simulink model "Fbridge_sim"  (R2023a)
settings: Solver=VariableStepAuto  StartTime=0.0  StopTime=20  MaxStep=1e-4  RelTol=1e-4  EnableMultiTasking=on
undefined symbols (not defined in the file or in its folder): D
libraries: spsMosfetLib x12, simulink x5, spsDCVoltageSourceLib x3, spsDCMachineLib x2, spsSeriesRLCBranchLib x2, spspowerguiLib x2, spsControlledVoltageSourceLib x1
settings Model: Creator=The MathWorks, Inc.  LastModifiedBy=Admin
settings SolverCC: AlgebraicLoopSolver=TrustRegion
settings DataIOCC: LimitDataPoints=on  SaveFormat=Array  ReturnWorkspaceOutputs=off
settings OptimizationCC: ExpressionDepthLimit=2147483647  InitFltsAndDblsToZero=on  LifeSpan=inf
settings DebuggingCC: SaveWithParameterizedLinksMsg=none  UnderspecifiedInitializationDetection=Classic  MergeDetectMultiDrivingBlocksExec=none  SignalResolutionControl=TryResolveAllWithWarning  SolverPrmCheckMsg=warning  MultiTaskDSMMsg=warning  MultiTaskCondExecSysMsg=none  FcnCallInpInsideContextMsg=warning  UnconnectedInputMsg=warning  UnconnectedOutputMsg=warning  UnconnectedLineMsg=warning  StateNameClashWarn=warning  SFUnexpectedBacktrackingDiag=warning  SFNoUnconditionalDefaultTransitionDiag=warning  SFExecutionAtInitializationDiag=none  ArithmeticOperatorsInVariantConditions=warning
settings HardwareCC: ProdBitPerPointer=32  ProdBitPerSizeT=32  ProdBitPerPtrDiffT=32  ProdLargestAtomicFloat=None  ProdIntDivRoundTo=Undefined  ProdEndianess=Unspecified  ProdWordSize=32  ProdHWDeviceType=32-bit Generic
settings ModelReferenceCC: EnableRefExpFcnMdlSchedulingChecks=on  PropagateSignalLabelsOutOfModel=off
settings SFSimCC: SimUseLocalCustomCode=off  CustomCodeUndefinedFunction=UseInterfaceOnly
settings RTWCC: RTWUseLocalCustomCode=off  DLArmComputeVersion=19.05
settings CodeAppCC: StateflowObjectComments=on
settings GRTTargetCC: TargetFcnLib=ansi_tfl_tmw.mat  TargetLangStandard=C89/C90 (ANSI)  CombineOutputUpdateFcns=off  GRTInterface=on
settings ConfigComp: CovMetricSettings=dw  CovSaveCumulativeToWorkspaceVar=on  CovSaveSingleToWorkspaceVar=on  CovExternalEMLEnable=off  CovSFcnEnable=off
settings SimscapeCC: SimscapeNormalizeSystem=off  SimscapeNominalValues={1, 'bar'; 1, 'cm^3/s'; 1, 'bar*kg/s'; 1, 'kJ/kg'; 1, 'kW'; }

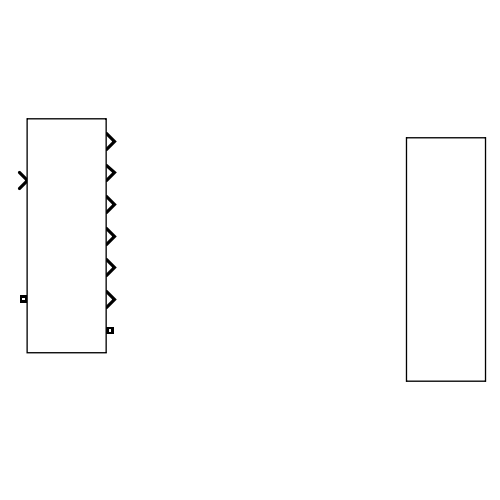
[thumbnail: Simulink's stored preview of the top-level diagram]
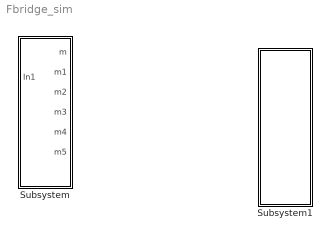
== system Fbridge_sim ==
  Subsystem : Subsystem
  Subsystem1 : Subsystem

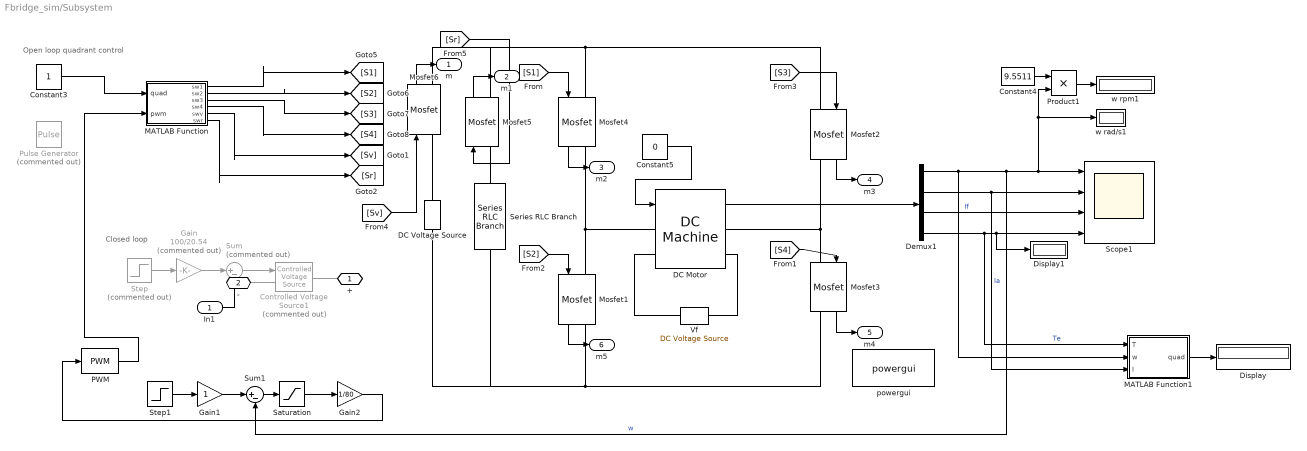
== system Fbridge_sim/Subsystem ==
  note: Open loop quadrant control
  note: Closed loop
  In1 : Inport
  Constant3 : Constant
  Constant4 : Constant  Value=9.5511
  Constant5 : Constant  Value=0
  Controlled Voltage Source1 : spsControlledVoltageSourceLib/Controlled Voltage Source  Commented=on  Initialize=on  Source_Type=DC  Amplitude=0  Phase=0  Frequency=0  Measurements=None
  DC Motor : spsDCMachineLib/DC Machine  PresetModel=No  MechanicalLoad=Torque TL  FieldType=Wound  ShowDetailedParameters=on  MeasurementBus=off  RLa=[2.581 0.028]  RLf=[2.02 0.128]  Laf=0.1  MachineConstant=Torque constant (N.m/A)  Ke=1.8  Kt=1.8  J=0.01  Bm=0.0006  Tf=0  w0=0  Ifinit=2.47524752475248  TsPowergui=0  TsBlock=-1
  DC Voltage Source : spsDCVoltageSourceLib/DC Voltage Source  Amplitude=80  Measurements=None
  Demux1 : Demux
  Display : Display
  Display1 : Display
  Gain : Gain  Commented=on  Gain=100/20.54
  Gain1 : Gain
  Gain2 : Gain  Gain=1/80
  MATLAB Function : MATLAB Function  TreatAsAtomicUnit=on
  MATLAB Function1 : MATLAB Function  TreatAsAtomicUnit=on
  Mosfet{1..6} (6 alike) : spsMosfetLib/Mosfet  Ron=0.1  Lon=0  Rd=0.01  Vfd=0  IC=0  Rs=1e5  Cs=inf  Measurements=on
  PWM : simulink/Discontinuities/PWM  DisableCoverage=on  Period=0.0001  InitialDelay=0  DisallowZeroDutyCycle=off  RunAtFixedTimeIntervals=off  SampleTime=0.1
  Product1 : Product
  Pulse Generator : DiscretePulseGenerator  Commented=on  PulseType=Time based  Period=0.0001  PulseWidth=D
  Saturation : Saturate  UpperLimit=80  LowerLimit=0
  Scope1 : Scope  NumInputPorts=4
  Series RLC Branch : spsSeriesRLCBranchLib/Series RLC Branch  LConnTagsString=__new0  RConnTagsString=__new0  BranchType=R  Resistance=10  Inductance=1e-3  SetiL0=off  InitialCurrent=0  Capacitance=1e-6  Setx0=off  InitialVoltage=0  Measurements=None
  Step : Step  Commented=on  After=100  SampleTime=0
  Step1 : Step  After=200  SampleTime=0
  Sum : Sum  Commented=on  Inputs=|+-
  Sum1 : Sum  Inputs=|+-
  Vf : spsDCVoltageSourceLib/DC Voltage Source  Amplitude=5  Measurements=None
  powergui : spspowerguiLib/powergui  SimulationMode=Discrete  SampleTime=20e-6  frequency=60  Iterations=50  frequencyindice=0  Pbase=100e6  ErrMax=1e-4  UnitsV=kV  UnitsW=MW  buscounter=0  FunctionMessages=off  echomessages=off  EnableUseOfTLC=off  CurrentSourceSwitches=off  DisableSnubberDevices=off  DisableRonSwitches=off  DisableVfSwitches=off  DisplayEquations=off  AutomaticDiscreteSolvers=off  SolverType=Tustin/Backward Euler (TBE)  Interpol=off  ExternalGateDelay=off  methode=off  Ts=100  x0status=blocks  SPID=on  SwTol=0  HookPort=off  NonlinearTolerance=1e-4  nMaxIteration=100  ContinueOnMaxIteration=off  RestoreLinks=warning  ResistiveCurrentMeasurement=off  Frange=[0:2:500]  Ylog=off  Xlog=on  ShowGrid=off  save=off  variable=ZData  structure=0  ZoomFFT=on  StartTime=0.0  cycles=1  DisplayStyle=1  fundamental=60  FreqAxis=off  MaxFrequency=1000  frequencyindicesteady=1  RmsSteady=1  display=off
  w rad/s1 : Display
  w rpm1 : Display
  + : PMIOPort  Side=Right
  - : PMIOPort  Port=2  Side=Left
  m : Outport
  m1 : Outport  Port=2
  m2 : Outport  Port=3
  m3 : Outport  Port=4
  m4 : Outport  Port=5
  m5 : Outport  Port=6
  wires:
  PWM/1 -> MATLAB Function/2(pwm)
  [S4] -> Mosfet3/1
  Mosfet4/1 -> m2/1
  MATLAB Function/1(sw1) -> [S1]
  Gain/1 -> Sum/1
  Demux1/3 -> Scope1/3  "If"
  Demux1/2 -> MATLAB Function1/3(I), Scope1/2  "Ia"
  Demux1/1 -> MATLAB Function1/2(w), Sum1/2, Scope1/1, Product1/2, w rad/s1/1  "w"
  DC Motor/1 -> Demux1/1
  Saturation/1 -> Gain2/1
  [Sr] -> Mosfet5/1
  [S1] -> Mosfet4/1
  In1/1 -> Sum/2
  Demux1/4 -> MATLAB Function1/1(T), Display1/1, Scope1/4  "Te"
  Mosfet3/1 -> m4/1
  Mosfet6/1 -> m/1
  [Sv] -> Mosfet6/1
  [S3] -> Mosfet2/1
  Sum/1 -> Controlled Voltage Source1/1
  [S2] -> Mosfet1/1
  Constant4/1 -> Product1/1
  Constant5/1 -> DC Motor/1
  MATLAB Function/3(sw3) -> [S3]
  Constant3/1 -> MATLAB Function/1(quad)
  Step1/1 -> Gain1/1
  MATLAB Function1/1(quad) -> Display/1
  MATLAB Function/5(swv) -> [Sv]
  MATLAB Function/6(swr) -> [Sr]
  MATLAB Function/2(sw2) -> [S2]
  MATLAB Function/4(sw4) -> [S4]
  Product1/1 -> w rpm1/1
  Sum1/1 -> Saturation/1
  Gain2/1 -> PWM/1
  Step/1 -> Gain/1
  Gain1/1 -> Sum1/1
  Mosfet1/1 -> m5/1
  Mosfet5/1 -> m1/1
  Mosfet2/1 -> m3/1
  connections:
  Mosfet4/LConn1 -- Mosfet5/RConn1 -- Mosfet6/RConn1 -- Mosfet2/LConn1
  Series RLC Branch/LConn1 -- Mosfet5/LConn1
  Mosfet4/RConn1 -- DC Motor/LConn1 -- Mosfet1/LConn1
  Controlled Voltage Source1/LConn1 -- -/RConn1
  DC Motor/RConn2 -- Vf/LConn1
  Mosfet6/LConn1 -- DC Voltage Source/RConn1
  Mosfet1/RConn1 -- Series RLC Branch/RConn1 -- DC Voltage Source/LConn1 -- Mosfet3/RConn1
  DC Motor/LConn2 -- Vf/RConn1
  DC Motor/RConn1 -- Mosfet3/LConn1 -- Mosfet2/RConn1
  Controlled Voltage Source1/RConn1 -- +/RConn1

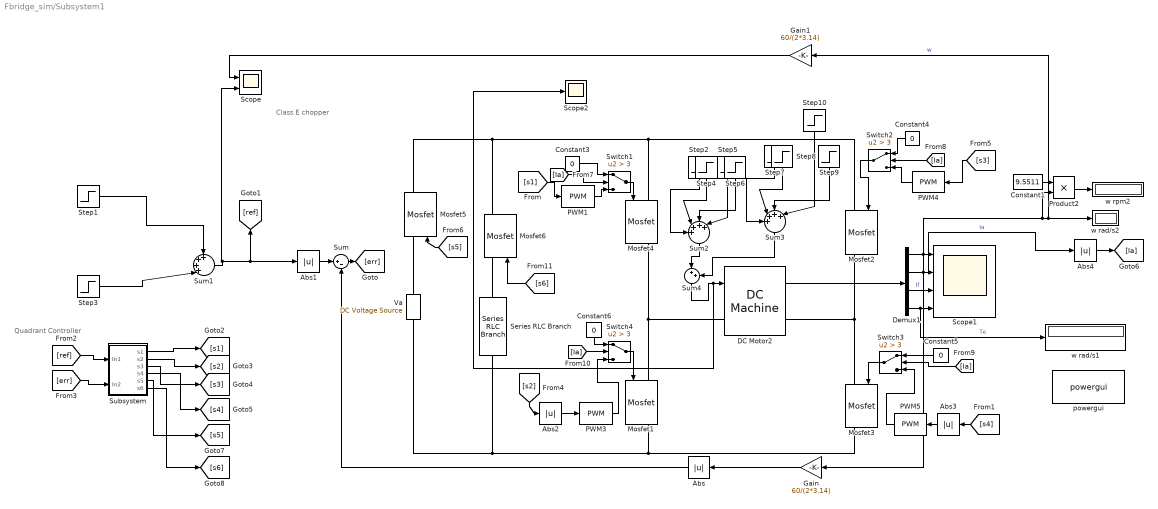
== system Fbridge_sim/Subsystem1 ==
  note: Quadrant Controller
  note: Class E chopper
  Abs{,1..4} (5 alike) : Abs  SaturateOnIntegerOverflow=off
  Constant1 : Constant  Value=9.5511
  Constant{3..6} (4 alike) : Constant  Value=0
  DC Motor2 : spsDCMachineLib/DC Machine  PresetModel=No  MechanicalLoad=Torque TL  FieldType=Permanent magnet  ShowDetailedParameters=on  MeasurementBus=off  RLa=[3 0.05]  RLf=[2.02 0.128]  Laf=0.1  MachineConstant=Back-emf constant (V/rpm)  Ke=0.029  Kt=0.27  J=0.012  Bm=0.0006  Tf=0.0958  w0=0  Ifinit=2.47524752475248  TsPowergui=0  TsBlock=-1
  Demux1 : Demux
  Gain : Gain  Gain=60/(2*3.14)
  Gain1 : Gain  Gain=60/(2*3.14)
  Mosfet{1..6} (6 alike) : spsMosfetLib/Mosfet  Ron=0.1  Lon=0  Rd=0.01  Vfd=0  IC=0  Rs=1e5  Cs=inf  Measurements=on
  PWM1 : simulink/Discontinuities/PWM  DisableCoverage=on  Period=1e-4  InitialDelay=0  DisallowZeroDutyCycle=off  RunAtFixedTimeIntervals=off  SampleTime=0.1
  PWM3 : simulink/Discontinuities/PWM  DisableCoverage=on  Period=5e-4  InitialDelay=0  DisallowZeroDutyCycle=off  RunAtFixedTimeIntervals=off  SampleTime=0.1
  PWM4 : simulink/Discontinuities/PWM  DisableCoverage=on  Period=1e-4  InitialDelay=0  DisallowZeroDutyCycle=off  RunAtFixedTimeIntervals=off  SampleTime=0.1
  PWM5 : simulink/Discontinuities/PWM  DisableCoverage=on  Period=5e-4  InitialDelay=0  DisallowZeroDutyCycle=off  RunAtFixedTimeIntervals=off  SampleTime=0.1
  Product2 : Product
  Scope : Scope  NumInputPorts=2
  Scope1 : Scope  NumInputPorts=4
  Scope2 : Scope
  Series RLC Branch : spsSeriesRLCBranchLib/Series RLC Branch  LConnTagsString=__new0  RConnTagsString=__new0  BranchType=R  Resistance=20  Inductance=1e-3  SetiL0=off  InitialCurrent=0  Capacitance=1e-6  Setx0=off  InitialVoltage=0  Measurements=None
  Step1 : Step  After=1000  SampleTime=0
  Step10 : Step  Time=17  After=-0.1  SampleTime=0
  Step2 : Step  Time=3  After=0.1  SampleTime=0
  Step3 : Step  Time=9  After=-2000  SampleTime=0
  Step4 : Step  Time=5  After=0.1  SampleTime=0
  Step5 : Step  Time=7  After=0.1  SampleTime=0
  Step6 : Step  Time=8  After=-0.3  SampleTime=0
  Step7 : Step  Time=12  After=-0.1  SampleTime=0
  Step8 : Step  Time=15  After=-0.1  SampleTime=0
  Step9 : Step  Time=18  After=+0.3  SampleTime=0
  Subsystem : Subsystem
  Sum : Sum  Inputs=|+-
  Sum1 : Sum  Inputs=++++|
  Sum2 : Sum  Inputs=++++|
  Sum3 : Sum  Inputs=++++|
  Sum4 : Sum  Inputs=|++
  Switch{1..4} (4 alike) : Switch  Criteria=u2 > Threshold  Threshold=3  SaturateOnIntegerOverflow=off  InputSameDT=off
  Va : spsDCVoltageSourceLib/DC Voltage Source  Amplitude=85  Measurements=None
  powergui : spspowerguiLib/powergui  SimulationMode=Discrete  SampleTime=20e-6  frequency=60  Iterations=50  frequencyindice=0  Pbase=100e6  ErrMax=1e-4  UnitsV=kV  UnitsW=MW  buscounter=0  FunctionMessages=off  echomessages=off  EnableUseOfTLC=off  CurrentSourceSwitches=off  DisableSnubberDevices=off  DisableRonSwitches=off  DisableVfSwitches=off  DisplayEquations=off  AutomaticDiscreteSolvers=off  SolverType=Tustin/Backward Euler (TBE)  Interpol=off  ExternalGateDelay=off  methode=off  Ts=100  x0status=blocks  SPID=on  SwTol=0  HookPort=off  NonlinearTolerance=1e-4  nMaxIteration=100  ContinueOnMaxIteration=off  RestoreLinks=warning  ResistiveCurrentMeasurement=off  Frange=[0:2:500]  Ylog=off  Xlog=on  ShowGrid=off  save=off  variable=ZData  structure=0  ZoomFFT=on  StartTime=0.0  cycles=1  DisplayStyle=1  fundamental=60  FreqAxis=off  MaxFrequency=1000  frequencyindicesteady=1  RmsSteady=1  display=off
  w rad/s1 : Display
  w rad/s2 : Display
  w rpm2 : Display
  wires:
  Demux1/4 -> w rad/s1/1, Scope1/4  "Te"
  DC Motor2/1 -> Demux1/1
  Demux1/2 -> Abs4/1, Scope1/2  "Ia"
  Demux1/3 -> Scope1/3  "If"
  Demux1/1 -> Gain1/1, w rad/s2/1, Product2/2, Gain/1, Scope1/1  "w"
  Constant1/1 -> Product2/1
  Product2/1 -> w rpm2/1
  [s2] -> Abs2/1
  [s3] -> PWM4/1
  Abs1/1 -> Sum/1
  [s1] -> PWM1/1
  Sum/1 -> [err]
  Subsystem/1(s1) -> [s1]
  Subsystem/2(s2) -> [s2]
  Subsystem/4(s4) -> [s4]
  Subsystem/3(s3) -> [s3]
  Step1/1 -> Sum1/1
  Sum1/1 -> Abs1/1, [ref], Scope/2
  [ref] -> Subsystem/1(In1)
  [err] -> Subsystem/2(In2)
  Abs2/1 -> PWM3/1
  Abs3/1 -> PWM5/1
  [s4] -> Abs3/1
  Step3/1 -> Sum1/4
  PWM1/1 -> Switch1/3
  Switch1/1 -> Mosfet4/1
  [Ia] -> Switch1/2
  Constant3/1 -> Switch1/1
  Gain/1 -> Abs/1
  Abs4/1 -> [Ia]
  PWM4/1 -> Switch2/3
  Constant4/1 -> Switch2/1
  [Ia] -> Switch2/2
  Switch2/1 -> Mosfet2/1
  Switch3/1 -> Mosfet3/1
  Constant5/1 -> Switch3/1
  [Ia] -> Switch3/2
  PWM5/1 -> Switch3/3
  PWM3/1 -> Switch4/3
  Constant6/1 -> Switch4/1
  [Ia] -> Switch4/2
  Switch4/1 -> Mosfet1/1
  [s5] -> Mosfet5/1
  Subsystem/5(s5) -> [s5]
  [s6] -> Mosfet6/1
  Gain1/1 -> Scope/1
  Abs/1 -> Sum/2
  Subsystem/6(s6) -> [s6]
  Step2/1 -> Sum2/1
  Step4/1 -> Sum2/2
  Step5/1 -> Sum2/4
  Step6/1 -> Sum2/3
  Sum2/1 -> Sum4/1
  Sum3/1 -> Sum4/2
  Sum4/1 -> Scope2/1, DC Motor2/1
  Step9/1 -> Sum3/3
  Step10/1 -> Sum3/4
  Step8/1 -> Sum3/2
  Step7/1 -> Sum3/1
  connections:
  Mosfet2/RConn1 -- Mosfet3/LConn1 -- DC Motor2/RConn1
  Mosfet4/RConn1 -- Mosfet1/LConn1 -- DC Motor2/LConn1
  Mosfet3/RConn1 -- Series RLC Branch/RConn1 -- Va/LConn1 -- Mosfet1/RConn1
  Mosfet4/LConn1 -- Mosfet5/RConn1 -- Mosfet6/RConn1 -- Mosfet2/LConn1
  Mosfet5/LConn1 -- Va/RConn1
  Mosfet6/LConn1 -- Series RLC Branch/LConn1

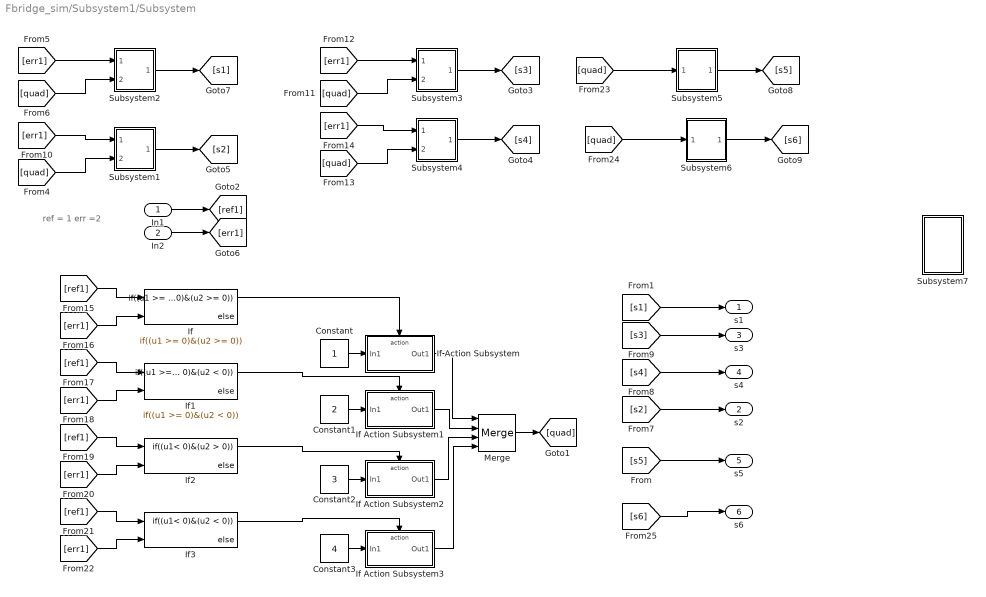
== system Fbridge_sim/Subsystem1/Subsystem ==
  note: ref = 1
      | err =2
  In1 : Inport
  In2 : Inport  Port=2
  Constant : Constant
  Constant1 : Constant  Value=2
  Constant2 : Constant  Value=3
  Constant3 : Constant  Value=4
  If : If  NumInputs=2  IfExpression=(u1 >= 0)&(u2 >= 0)
  If Action Subsystem : Subsystem  TreatAsAtomicUnit=on
  If Action Subsystem1 : Subsystem  TreatAsAtomicUnit=on
  If Action Subsystem2 : Subsystem  TreatAsAtomicUnit=on
  If Action Subsystem3 : Subsystem  TreatAsAtomicUnit=on
  If1 : If  NumInputs=2  IfExpression=(u1 >= 0)&(u2 < 0)
  If2 : If  NumInputs=2  IfExpression=(u1< 0)&(u2 > 0)
  If3 : If  NumInputs=2  IfExpression=(u1< 0)&(u2 < 0)
  Merge : Merge  Inputs=4
  Subsystem1 : Subsystem
  Subsystem2 : Subsystem
  Subsystem3 : Subsystem
  Subsystem4 : Subsystem
  Subsystem5 : Subsystem
  Subsystem6 : Subsystem
  Subsystem7 : Subsystem
  s1 : Outport
  s2 : Outport  Port=2
  s3 : Outport  Port=3
  s4 : Outport  Port=4
  s5 : Outport  Port=5
  s6 : Outport  Port=6
  wires:
  In1/1 -> [ref1]
  [s1] -> s1/1
  In2/1 -> [err1]
  [err1] -> Subsystem1/1(In1)
  [quad] -> Subsystem1/2(In2)
  Subsystem1/1(Out1) -> [s2]
  Subsystem2/1(Out1) -> [s1]
  [quad] -> Subsystem2/2(In2)
  [err1] -> Subsystem2/1(In1)
  [s3] -> s3/1
  [err1] -> Subsystem3/1(In1)
  [quad] -> Subsystem3/2(In2)
  Subsystem3/1(Out1) -> [s3]
  Subsystem4/1(Out1) -> [s4]
  [quad] -> Subsystem4/2(In2)
  [err1] -> Subsystem4/1(In1)
  [s2] -> s2/1
  [s4] -> s4/1
  [ref1] -> If/1
  [err1] -> If/2
  If/1 -> If Action Subsystem/Action
  If Action Subsystem/1(Out1) -> Merge/1
  Constant/1 -> If Action Subsystem/1(In1)
  Merge/1 -> [quad]
  [err1] -> If1/2
  [ref1] -> If1/1
  Constant1/1 -> If Action Subsystem1/1(In1)
  If Action Subsystem1/1(Out1) -> Merge/2
  If1/1 -> If Action Subsystem1/Action
  If2/1 -> If Action Subsystem2/Action
  [ref1] -> If2/1
  [err1] -> If2/2
  [err1] -> If3/2
  [ref1] -> If3/1
  If3/1 -> If Action Subsystem3/Action
  Constant2/1 -> If Action Subsystem2/1(In1)
  Constant3/1 -> If Action Subsystem3/1(In1)
  If Action Subsystem2/1(Out1) -> Merge/3
  If Action Subsystem3/1(Out1) -> Merge/4
  Subsystem5/1(Out1) -> [s5]
  [quad] -> Subsystem5/1(In2)
  [s5] -> s5/1
  [s6] -> s6/1
  [quad] -> Subsystem6/1(In2)
  Subsystem6/1(Out1) -> [s6]

== system Fbridge_sim/Subsystem1/Subsystem/If Action Subsystem ==
  In1 : Inport
  Action Port : ActionPort  ActionPortLabel=if((u1 >= 0)&(u2 >= 0))
  Out1 : Outport
  wires:
  In1/1 -> Out1/1

== system Fbridge_sim/Subsystem1/Subsystem/If Action Subsystem1 ==
  In1 : Inport
  Action Port : ActionPort  ActionPortLabel=if((u1 >= 0)&(u2 < 0))
  Out1 : Outport
  wires:
  In1/1 -> Out1/1

== system Fbridge_sim/Subsystem1/Subsystem/If Action Subsystem2 ==
  In1 : Inport
  Action Port : ActionPort  ActionPortLabel=if((u1< 0)&(u2 > 0))
  Out1 : Outport
  wires:
  In1/1 -> Out1/1

== system Fbridge_sim/Subsystem1/Subsystem/If Action Subsystem3 ==
  In1 : Inport
  Action Port : ActionPort  ActionPortLabel=if((u1< 0)&(u2 < 0))
  Out1 : Outport
  wires:
  In1/1 -> Out1/1

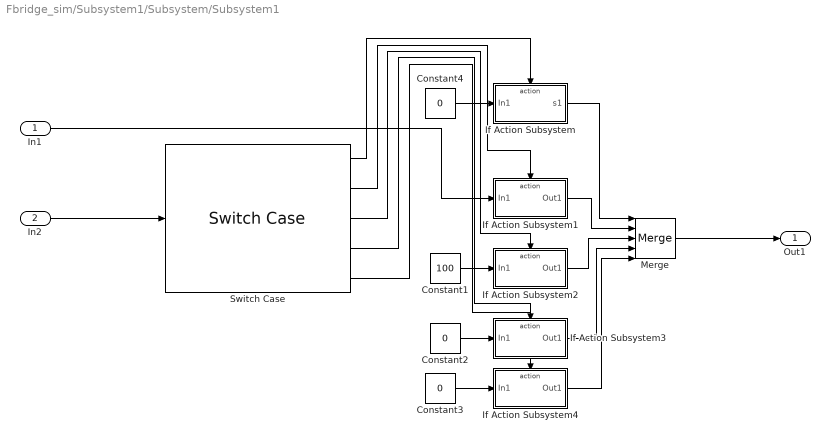
== system Fbridge_sim/Subsystem1/Subsystem/Subsystem1 ==
  In1 : Inport
  In2 : Inport  Port=2
  Constant1 : Constant  Value=100
  Constant2 : Constant  Value=0
  Constant3 : Constant  Value=0
  Constant4 : Constant  Value=0
  If Action Subsystem : Subsystem  TreatAsAtomicUnit=on
      settings: LibrarySourceBlock=|
      | hdlsllib/Ports &
      | Subsystems/If Action
      | Subsystem
  If Action Subsystem1 : Subsystem  TreatAsAtomicUnit=on
      settings: LibrarySourceBlock=|
      | hdlsllib/Ports &
      | Subsystems/If Action
      | Subsystem
  If Action Subsystem2 : Subsystem  TreatAsAtomicUnit=on
      settings: LibrarySourceBlock=|
      | hdlsllib/Ports &
      | Subsystems/If Action
      | Subsystem
  If Action Subsystem3 : Subsystem  TreatAsAtomicUnit=on
      settings: LibrarySourceBlock=|
      | hdlsllib/Ports &
      | Subsystems/If Action
      | Subsystem
  If Action Subsystem4 : Subsystem  TreatAsAtomicUnit=on
      settings: LibrarySourceBlock=|
      | hdlsllib/Ports &
      | Subsystems/If Action
      | Subsystem
  Merge : Merge  Inputs=5
  Switch Case : SwitchCase  CaseConditions={1,2,3,4}
  Out1 : Outport
  wires:
  If Action Subsystem4/1(Out1) -> Merge/5
  Switch Case/2 -> If Action Subsystem1/Action
  Switch Case/4 -> If Action Subsystem3/Action
  Switch Case/1 -> If Action Subsystem/Action
  In1/1 -> If Action Subsystem1/1(In1)
  Switch Case/3 -> If Action Subsystem2/Action
  Switch Case/5 -> If Action Subsystem4/Action
  If Action Subsystem1/1(Out1) -> Merge/2
  If Action Subsystem/1(s1) -> Merge/1
  If Action Subsystem2/1(Out1) -> Merge/3
  Constant1/1 -> If Action Subsystem2/1(In1)
  Constant2/1 -> If Action Subsystem3/1(In1)
  If Action Subsystem3/1(Out1) -> Merge/4
  Constant3/1 -> If Action Subsystem4/1(In1)
  In2/1 -> Switch Case/1
  Merge/1 -> Out1/1
  Constant4/1 -> If Action Subsystem/1(In1)

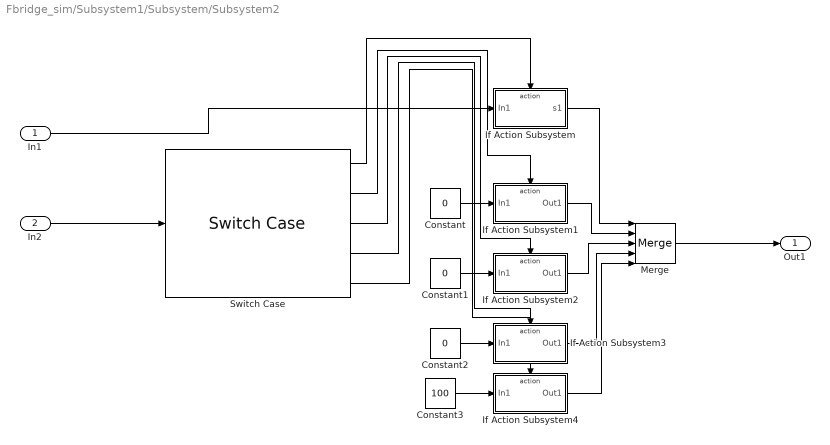
== system Fbridge_sim/Subsystem1/Subsystem/Subsystem2 ==
  In1 : Inport
  In2 : Inport  Port=2
  Constant : Constant  Value=0
  Constant1 : Constant  Value=0
  Constant2 : Constant  Value=0
  Constant3 : Constant  Value=100
  If Action Subsystem : Subsystem  TreatAsAtomicUnit=on
      settings: LibrarySourceBlock=|
      | hdlsllib/Ports &
      | Subsystems/If Action
      | Subsystem
  If Action Subsystem1 : Subsystem  TreatAsAtomicUnit=on
      settings: LibrarySourceBlock=|
      | hdlsllib/Ports &
      | Subsystems/If Action
      | Subsystem
  If Action Subsystem2 : Subsystem  TreatAsAtomicUnit=on
      settings: LibrarySourceBlock=|
      | hdlsllib/Ports &
      | Subsystems/If Action
      | Subsystem
  If Action Subsystem3 : Subsystem  TreatAsAtomicUnit=on
      settings: LibrarySourceBlock=|
      | hdlsllib/Ports &
      | Subsystems/If Action
      | Subsystem
  If Action Subsystem4 : Subsystem  TreatAsAtomicUnit=on
      settings: LibrarySourceBlock=|
      | hdlsllib/Ports &
      | Subsystems/If Action
      | Subsystem
  Merge : Merge  Inputs=5
  Switch Case : SwitchCase  CaseConditions={1,2,3,4}
  Out1 : Outport
  wires:
  Merge/1 -> Out1/1
  In1/1 -> If Action Subsystem/1(In1)
  In2/1 -> Switch Case/1
  Constant3/1 -> If Action Subsystem4/1(In1)
  If Action Subsystem3/1(Out1) -> Merge/4
  Constant2/1 -> If Action Subsystem3/1(In1)
  Constant1/1 -> If Action Subsystem2/1(In1)
  If Action Subsystem2/1(Out1) -> Merge/3
  If Action Subsystem/1(s1) -> Merge/1
  If Action Subsystem1/1(Out1) -> Merge/2
  Switch Case/5 -> If Action Subsystem4/Action
  Switch Case/3 -> If Action Subsystem2/Action
  Constant/1 -> If Action Subsystem1/1(In1)
  Switch Case/1 -> If Action Subsystem/Action
  Switch Case/4 -> If Action Subsystem3/Action
  Switch Case/2 -> If Action Subsystem1/Action
  If Action Subsystem4/1(Out1) -> Merge/5

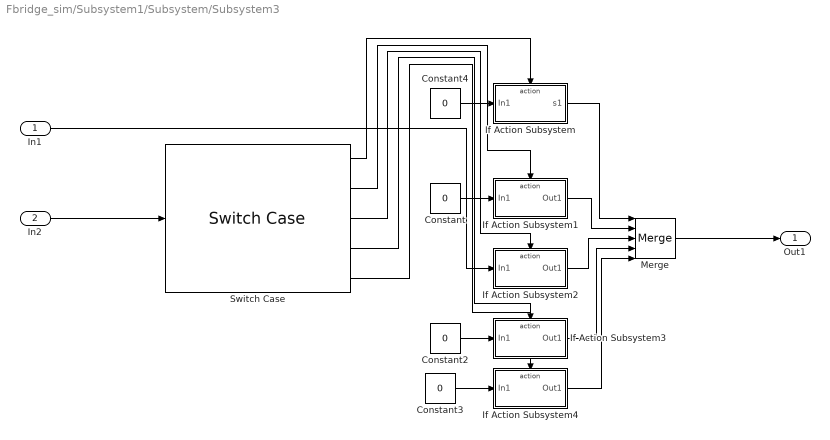
== system Fbridge_sim/Subsystem1/Subsystem/Subsystem3 ==
  In1 : Inport
  In2 : Inport  Port=2
  Constant{,2..4} (4 alike) : Constant  Value=0
  If Action Subsystem : Subsystem  TreatAsAtomicUnit=on
      settings: LibrarySourceBlock=|
      | hdlsllib/Ports &
      | Subsystems/If Action
      | Subsystem
  If Action Subsystem1 : Subsystem  TreatAsAtomicUnit=on
      settings: LibrarySourceBlock=|
      | hdlsllib/Ports &
      | Subsystems/If Action
      | Subsystem
  If Action Subsystem2 : Subsystem  TreatAsAtomicUnit=on
      settings: LibrarySourceBlock=|
      | hdlsllib/Ports &
      | Subsystems/If Action
      | Subsystem
  If Action Subsystem3 : Subsystem  TreatAsAtomicUnit=on
      settings: LibrarySourceBlock=|
      | hdlsllib/Ports &
      | Subsystems/If Action
      | Subsystem
  If Action Subsystem4 : Subsystem  TreatAsAtomicUnit=on
      settings: LibrarySourceBlock=|
      | hdlsllib/Ports &
      | Subsystems/If Action
      | Subsystem
  Merge : Merge  Inputs=5
  Switch Case : SwitchCase  CaseConditions={1,2,3,4}
  Out1 : Outport
  wires:
  If Action Subsystem4/1(Out1) -> Merge/5
  Switch Case/2 -> If Action Subsystem1/Action
  Switch Case/4 -> If Action Subsystem3/Action
  Switch Case/1 -> If Action Subsystem/Action
  Constant/1 -> If Action Subsystem1/1(In1)
  Switch Case/3 -> If Action Subsystem2/Action
  Switch Case/5 -> If Action Subsystem4/Action
  If Action Subsystem1/1(Out1) -> Merge/2
  If Action Subsystem/1(s1) -> Merge/1
  If Action Subsystem2/1(Out1) -> Merge/3
  In1/1 -> If Action Subsystem2/1(In1)
  Constant2/1 -> If Action Subsystem3/1(In1)
  If Action Subsystem3/1(Out1) -> Merge/4
  Constant3/1 -> If Action Subsystem4/1(In1)
  In2/1 -> Switch Case/1
  Merge/1 -> Out1/1
  Constant4/1 -> If Action Subsystem/1(In1)

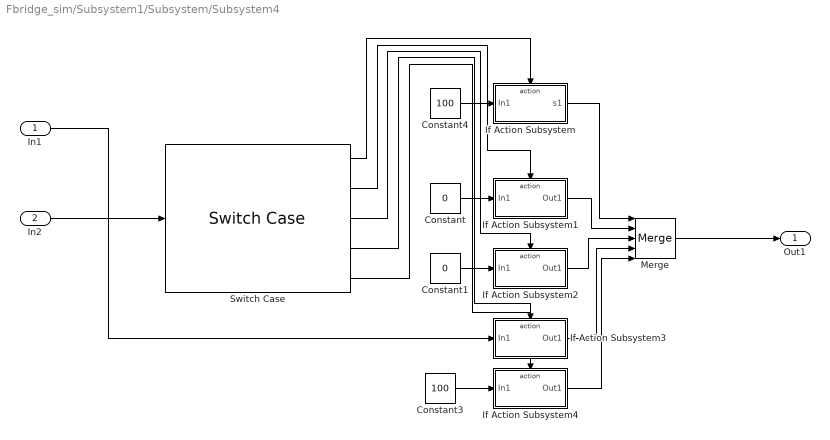
== system Fbridge_sim/Subsystem1/Subsystem/Subsystem4 ==
  In1 : Inport
  In2 : Inport  Port=2
  Constant : Constant  Value=0
  Constant1 : Constant  Value=0
  Constant3 : Constant  Value=100
  Constant4 : Constant  Value=100
  If Action Subsystem : Subsystem  TreatAsAtomicUnit=on
      settings: LibrarySourceBlock=|
      | hdlsllib/Ports &
      | Subsystems/If Action
      | Subsystem
  If Action Subsystem1 : Subsystem  TreatAsAtomicUnit=on
      settings: LibrarySourceBlock=|
      | hdlsllib/Ports &
      | Subsystems/If Action
      | Subsystem
  If Action Subsystem2 : Subsystem  TreatAsAtomicUnit=on
      settings: LibrarySourceBlock=|
      | hdlsllib/Ports &
      | Subsystems/If Action
      | Subsystem
  If Action Subsystem3 : Subsystem  TreatAsAtomicUnit=on
      settings: LibrarySourceBlock=|
      | hdlsllib/Ports &
      | Subsystems/If Action
      | Subsystem
  If Action Subsystem4 : Subsystem  TreatAsAtomicUnit=on
      settings: LibrarySourceBlock=|
      | hdlsllib/Ports &
      | Subsystems/If Action
      | Subsystem
  Merge : Merge  Inputs=5
  Switch Case : SwitchCase  CaseConditions={1,2,3,4}
  Out1 : Outport
  wires:
  Merge/1 -> Out1/1
  In2/1 -> Switch Case/1
  Constant3/1 -> If Action Subsystem4/1(In1)
  If Action Subsystem3/1(Out1) -> Merge/4
  In1/1 -> If Action Subsystem3/1(In1)
  Constant1/1 -> If Action Subsystem2/1(In1)
  If Action Subsystem2/1(Out1) -> Merge/3
  If Action Subsystem/1(s1) -> Merge/1
  If Action Subsystem1/1(Out1) -> Merge/2
  Switch Case/5 -> If Action Subsystem4/Action
  Switch Case/3 -> If Action Subsystem2/Action
  Constant/1 -> If Action Subsystem1/1(In1)
  Switch Case/1 -> If Action Subsystem/Action
  Switch Case/4 -> If Action Subsystem3/Action
  Switch Case/2 -> If Action Subsystem1/Action
  If Action Subsystem4/1(Out1) -> Merge/5
  Constant4/1 -> If Action Subsystem/1(In1)

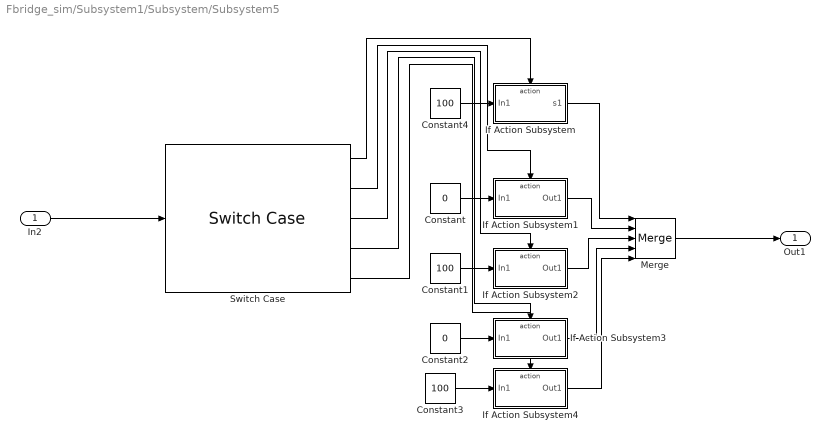
== system Fbridge_sim/Subsystem1/Subsystem/Subsystem5 ==
  In2 : Inport
  Constant : Constant  Value=0
  Constant1 : Constant  Value=100
  Constant2 : Constant  Value=0
  Constant3 : Constant  Value=100
  Constant4 : Constant  Value=100
  If Action Subsystem : Subsystem  TreatAsAtomicUnit=on
      settings: LibrarySourceBlock=|
      | hdlsllib/Ports &
      | Subsystems/If Action
      | Subsystem
  If Action Subsystem1 : Subsystem  TreatAsAtomicUnit=on
      settings: LibrarySourceBlock=|
      | hdlsllib/Ports &
      | Subsystems/If Action
      | Subsystem
  If Action Subsystem2 : Subsystem  TreatAsAtomicUnit=on
      settings: LibrarySourceBlock=|
      | hdlsllib/Ports &
      | Subsystems/If Action
      | Subsystem
  If Action Subsystem3 : Subsystem  TreatAsAtomicUnit=on
      settings: LibrarySourceBlock=|
      | hdlsllib/Ports &
      | Subsystems/If Action
      | Subsystem
  If Action Subsystem4 : Subsystem  TreatAsAtomicUnit=on
      settings: LibrarySourceBlock=|
      | hdlsllib/Ports &
      | Subsystems/If Action
      | Subsystem
  Merge : Merge  Inputs=5
  Switch Case : SwitchCase  CaseConditions={1,2,3,4}
  Out1 : Outport
  wires:
  Constant4/1 -> If Action Subsystem/1(In1)
  Merge/1 -> Out1/1
  In2/1 -> Switch Case/1
  Constant3/1 -> If Action Subsystem4/1(In1)
  If Action Subsystem3/1(Out1) -> Merge/4
  Constant2/1 -> If Action Subsystem3/1(In1)
  If Action Subsystem2/1(Out1) -> Merge/3
  If Action Subsystem/1(s1) -> Merge/1
  If Action Subsystem1/1(Out1) -> Merge/2
  Switch Case/5 -> If Action Subsystem4/Action
  Switch Case/3 -> If Action Subsystem2/Action
  Constant/1 -> If Action Subsystem1/1(In1)
  Switch Case/1 -> If Action Subsystem/Action
  Switch Case/4 -> If Action Subsystem3/Action
  Switch Case/2 -> If Action Subsystem1/Action
  If Action Subsystem4/1(Out1) -> Merge/5
  Constant1/1 -> If Action Subsystem2/1(In1)

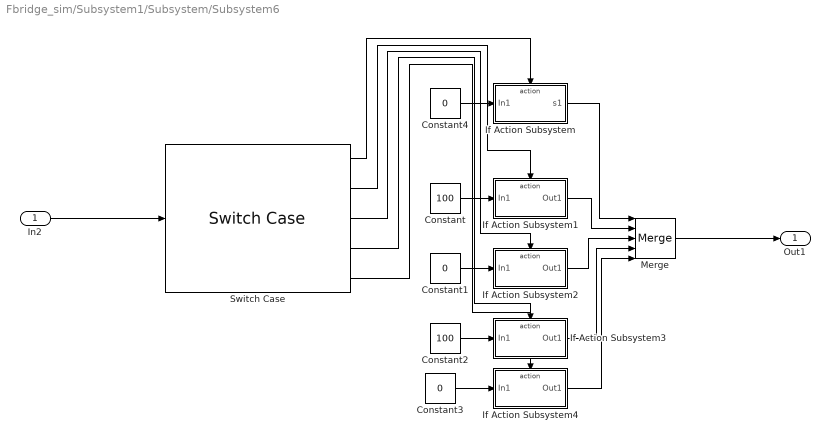
== system Fbridge_sim/Subsystem1/Subsystem/Subsystem6 ==
  In2 : Inport
  Constant : Constant  Value=100
  Constant1 : Constant  Value=0
  Constant2 : Constant  Value=100
  Constant3 : Constant  Value=0
  Constant4 : Constant  Value=0
  If Action Subsystem : Subsystem  TreatAsAtomicUnit=on
      settings: LibrarySourceBlock=|
      | hdlsllib/Ports &
      | Subsystems/If Action
      | Subsystem
  If Action Subsystem1 : Subsystem  TreatAsAtomicUnit=on
      settings: LibrarySourceBlock=|
      | hdlsllib/Ports &
      | Subsystems/If Action
      | Subsystem
  If Action Subsystem2 : Subsystem  TreatAsAtomicUnit=on
      settings: LibrarySourceBlock=|
      | hdlsllib/Ports &
      | Subsystems/If Action
      | Subsystem
  If Action Subsystem3 : Subsystem  TreatAsAtomicUnit=on
      settings: LibrarySourceBlock=|
      | hdlsllib/Ports &
      | Subsystems/If Action
      | Subsystem
  If Action Subsystem4 : Subsystem  TreatAsAtomicUnit=on
      settings: LibrarySourceBlock=|
      | hdlsllib/Ports &
      | Subsystems/If Action
      | Subsystem
  Merge : Merge  Inputs=5
  Switch Case : SwitchCase  CaseConditions={1,2,3,4}
  Out1 : Outport
  wires:
  Constant1/1 -> If Action Subsystem2/1(In1)
  If Action Subsystem4/1(Out1) -> Merge/5
  Switch Case/2 -> If Action Subsystem1/Action
  Switch Case/4 -> If Action Subsystem3/Action
  Switch Case/1 -> If Action Subsystem/Action
  Constant/1 -> If Action Subsystem1/1(In1)
  Switch Case/3 -> If Action Subsystem2/Action
  Switch Case/5 -> If Action Subsystem4/Action
  If Action Subsystem1/1(Out1) -> Merge/2
  If Action Subsystem/1(s1) -> Merge/1
  If Action Subsystem2/1(Out1) -> Merge/3
  Constant2/1 -> If Action Subsystem3/1(In1)
  If Action Subsystem3/1(Out1) -> Merge/4
  Constant3/1 -> If Action Subsystem4/1(In1)
  In2/1 -> Switch Case/1
  Merge/1 -> Out1/1
  Constant4/1 -> If Action Subsystem/1(In1)

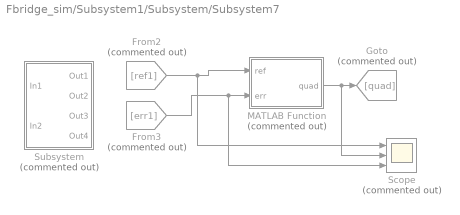
== system Fbridge_sim/Subsystem1/Subsystem/Subsystem7 ==
  From2 : From  Commented=on  GotoTag=ref1
  From3 : From  Commented=on  GotoTag=err1
  Goto : Goto  Commented=on  GotoTag=quad
  MATLAB Function : MATLAB Function  Commented=on  TreatAsAtomicUnit=on
  Scope : Scope  Commented=on  NumInputPorts=3
  Subsystem : Subsystem  Commented=on
  wires:
  From2/1 -> Scope/1, MATLAB Function/1(ref)
  MATLAB Function/1(quad) -> Scope/2, Goto/1
  From3/1 -> Scope/3, MATLAB Function/2(err)

== system Fbridge_sim/Subsystem1/Subsystem/Subsystem1/If Action Subsystem ==
  In1 : Inport
  Action Port : ActionPort  ActionPortLabel=case [ 1 ]:
  s1 : Outport
  wires:
  In1/1 -> s1/1

== system Fbridge_sim/Subsystem1/Subsystem/Subsystem1/If Action Subsystem1 ==
  In1 : Inport
  Action Port : ActionPort  ActionPortLabel=case [ 2 ]:
  Out1 : Outport
  wires:
  In1/1 -> Out1/1

== system Fbridge_sim/Subsystem1/Subsystem/Subsystem1/If Action Subsystem2 ==
  In1 : Inport
  Action Port : ActionPort  ActionPortLabel=case [ 3 ]:
  Out1 : Outport
  wires:
  In1/1 -> Out1/1

== system Fbridge_sim/Subsystem1/Subsystem/Subsystem1/If Action Subsystem3 ==
  In1 : Inport
  Action Port : ActionPort  ActionPortLabel=case [ 4 ]:
  Out1 : Outport
  wires:
  In1/1 -> Out1/1

== system Fbridge_sim/Subsystem1/Subsystem/Subsystem1/If Action Subsystem4 ==
  In1 : Inport
  Action Port : ActionPort  ActionPortLabel=default:
  Out1 : Outport
  wires:
  In1/1 -> Out1/1

== system Fbridge_sim/Subsystem1/Subsystem/Subsystem2/If Action Subsystem ==
  In1 : Inport
  Action Port : ActionPort  ActionPortLabel=case [ 1 ]:
  s1 : Outport
  wires:
  In1/1 -> s1/1

== system Fbridge_sim/Subsystem1/Subsystem/Subsystem2/If Action Subsystem1 ==
  In1 : Inport
  Action Port : ActionPort  ActionPortLabel=case [ 2 ]:
  Out1 : Outport
  wires:
  In1/1 -> Out1/1

== system Fbridge_sim/Subsystem1/Subsystem/Subsystem2/If Action Subsystem2 ==
  In1 : Inport
  Action Port : ActionPort  ActionPortLabel=case [ 3 ]:
  Out1 : Outport
  wires:
  In1/1 -> Out1/1

== system Fbridge_sim/Subsystem1/Subsystem/Subsystem2/If Action Subsystem3 ==
  In1 : Inport
  Action Port : ActionPort  ActionPortLabel=case [ 4 ]:
  Out1 : Outport
  wires:
  In1/1 -> Out1/1

== system Fbridge_sim/Subsystem1/Subsystem/Subsystem2/If Action Subsystem4 ==
  In1 : Inport
  Action Port : ActionPort  ActionPortLabel=default:
  Out1 : Outport
  wires:
  In1/1 -> Out1/1

== system Fbridge_sim/Subsystem1/Subsystem/Subsystem3/If Action Subsystem ==
  In1 : Inport
  Action Port : ActionPort  ActionPortLabel=case [ 1 ]:
  s1 : Outport
  wires:
  In1/1 -> s1/1

== system Fbridge_sim/Subsystem1/Subsystem/Subsystem3/If Action Subsystem1 ==
  In1 : Inport
  Action Port : ActionPort  ActionPortLabel=case [ 2 ]:
  Out1 : Outport
  wires:
  In1/1 -> Out1/1

== system Fbridge_sim/Subsystem1/Subsystem/Subsystem3/If Action Subsystem2 ==
  In1 : Inport
  Action Port : ActionPort  ActionPortLabel=case [ 3 ]:
  Out1 : Outport
  wires:
  In1/1 -> Out1/1

== system Fbridge_sim/Subsystem1/Subsystem/Subsystem3/If Action Subsystem3 ==
  In1 : Inport
  Action Port : ActionPort  ActionPortLabel=case [ 4 ]:
  Out1 : Outport
  wires:
  In1/1 -> Out1/1

== system Fbridge_sim/Subsystem1/Subsystem/Subsystem3/If Action Subsystem4 ==
  In1 : Inport
  Action Port : ActionPort  ActionPortLabel=default:
  Out1 : Outport
  wires:
  In1/1 -> Out1/1

== system Fbridge_sim/Subsystem1/Subsystem/Subsystem4/If Action Subsystem ==
  In1 : Inport
  Action Port : ActionPort  ActionPortLabel=case [ 1 ]:
  s1 : Outport
  wires:
  In1/1 -> s1/1

== system Fbridge_sim/Subsystem1/Subsystem/Subsystem4/If Action Subsystem1 ==
  In1 : Inport
  Action Port : ActionPort  ActionPortLabel=case [ 2 ]:
  Out1 : Outport
  wires:
  In1/1 -> Out1/1

== system Fbridge_sim/Subsystem1/Subsystem/Subsystem4/If Action Subsystem2 ==
  In1 : Inport
  Action Port : ActionPort  ActionPortLabel=case [ 3 ]:
  Out1 : Outport
  wires:
  In1/1 -> Out1/1

== system Fbridge_sim/Subsystem1/Subsystem/Subsystem4/If Action Subsystem3 ==
  In1 : Inport
  Action Port : ActionPort  ActionPortLabel=case [ 4 ]:
  Out1 : Outport
  wires:
  In1/1 -> Out1/1

== system Fbridge_sim/Subsystem1/Subsystem/Subsystem4/If Action Subsystem4 ==
  In1 : Inport
  Action Port : ActionPort  ActionPortLabel=default:
  Out1 : Outport
  wires:
  In1/1 -> Out1/1

== system Fbridge_sim/Subsystem1/Subsystem/Subsystem5/If Action Subsystem ==
  In1 : Inport
  Action Port : ActionPort  ActionPortLabel=case [ 1 ]:
  s1 : Outport
  wires:
  In1/1 -> s1/1

== system Fbridge_sim/Subsystem1/Subsystem/Subsystem5/If Action Subsystem1 ==
  In1 : Inport
  Action Port : ActionPort  ActionPortLabel=case [ 2 ]:
  Out1 : Outport
  wires:
  In1/1 -> Out1/1

== system Fbridge_sim/Subsystem1/Subsystem/Subsystem5/If Action Subsystem2 ==
  In1 : Inport
  Action Port : ActionPort  ActionPortLabel=case [ 3 ]:
  Out1 : Outport
  wires:
  In1/1 -> Out1/1

== system Fbridge_sim/Subsystem1/Subsystem/Subsystem5/If Action Subsystem3 ==
  In1 : Inport
  Action Port : ActionPort  ActionPortLabel=case [ 4 ]:
  Out1 : Outport
  wires:
  In1/1 -> Out1/1

== system Fbridge_sim/Subsystem1/Subsystem/Subsystem5/If Action Subsystem4 ==
  In1 : Inport
  Action Port : ActionPort  ActionPortLabel=default:
  Out1 : Outport
  wires:
  In1/1 -> Out1/1

== system Fbridge_sim/Subsystem1/Subsystem/Subsystem6/If Action Subsystem ==
  In1 : Inport
  Action Port : ActionPort  ActionPortLabel=case [ 1 ]:
  s1 : Outport
  wires:
  In1/1 -> s1/1

== system Fbridge_sim/Subsystem1/Subsystem/Subsystem6/If Action Subsystem1 ==
  In1 : Inport
  Action Port : ActionPort  ActionPortLabel=case [ 2 ]:
  Out1 : Outport
  wires:
  In1/1 -> Out1/1

== system Fbridge_sim/Subsystem1/Subsystem/Subsystem6/If Action Subsystem2 ==
  In1 : Inport
  Action Port : ActionPort  ActionPortLabel=case [ 3 ]:
  Out1 : Outport
  wires:
  In1/1 -> Out1/1

== system Fbridge_sim/Subsystem1/Subsystem/Subsystem6/If Action Subsystem3 ==
  In1 : Inport
  Action Port : ActionPort  ActionPortLabel=case [ 4 ]:
  Out1 : Outport
  wires:
  In1/1 -> Out1/1

== system Fbridge_sim/Subsystem1/Subsystem/Subsystem6/If Action Subsystem4 ==
  In1 : Inport
  Action Port : ActionPort  ActionPortLabel=default:
  Out1 : Outport
  wires:
  In1/1 -> Out1/1

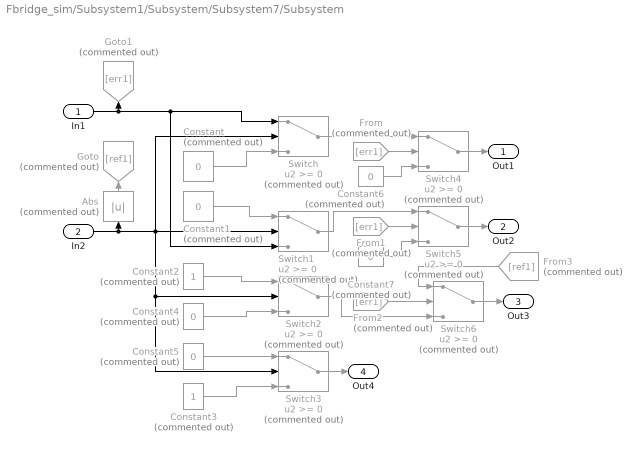
== system Fbridge_sim/Subsystem1/Subsystem/Subsystem7/Subsystem ==
  In1 : Inport
  In2 : Inport  Port=2
  Abs : Abs  Commented=on  SaturateOnIntegerOverflow=off
  Constant{,1,4..7} (6 alike) : Constant  Commented=on  Value=0
  Constant2 : Constant  Commented=on
  Constant3 : Constant  Commented=on
  From : From  Commented=on  GotoTag=err1
  From1 : From  Commented=on  GotoTag=err1
  From2 : From  Commented=on  GotoTag=err1
  From3 : From  Commented=on  GotoTag=ref1
  Goto : Goto  Commented=on  GotoTag=ref1
  Goto1 : Goto  Commented=on  GotoTag=err1
  Switch{,1..6} (7 alike) : Switch  Commented=on  SaturateOnIntegerOverflow=off  InputSameDT=off
  Out1 : Outport
  Out2 : Outport  Port=2
  Out3 : Outport  Port=3
  Out4 : Outport  Port=4
  wires:
  Constant1/1 -> Switch1/1
  In1/1 -> Goto1/1, Switch1/3, Switch/1
  Constant6/1 -> Switch4/3
  From2/1 -> Switch6/2
  Switch/1 -> Switch4/1
  Constant4/1 -> Switch2/3
  From/1 -> Switch4/2
  Switch4/1 -> Out1/1
  Switch1/1 -> Switch5/1
  Constant2/1 -> Switch2/1
  Switch6/1 -> Out3/1
  From3/1 -> Switch6/1
  From1/1 -> Switch5/2
  Switch2/1 -> Switch6/3
  Constant5/1 -> Switch3/1
  Constant7/1 -> Switch5/3
  Constant3/1 -> Switch3/3
  Abs/1 -> Goto/1
  Constant/1 -> Switch/3
  In2/1 -> Abs/1, Switch/2, Switch2/2, Switch3/2, Switch1/2
  Switch3/1 -> Out4/1
  Switch5/1 -> Out2/1

== matlab function Fbridge_sim/Subsystem/MATLAB Function1 ==
  data: T input; quad output; w input; I input
function quad = fcn(T,w,I)

if w>=0
    quad = 1;
else
    quad = 2;

end

== matlab function Fbridge_sim/Subsystem/MATLAB Function ==
  data: quad input; sw1 output; sw2 output; sw3 output; sw4 output; pwm input; swv output; swr output
function [sw1,sw2,sw3,sw4,swv,swr]= fcn(quad,pwm)

sw1=0;sw2=0;sw3=0; sw4=0; swv=1; swr=0; 

if (quad == 1)

    sw1=pwm;sw2=0;sw3=0; sw4=1; 
end

if (quad == 2)

    sw1=0;sw2=1;sw3=pwm; sw4=0; 
end
if (quad == 3)

    sw1=0;sw2=pwm;sw3=0; sw4=0; swv=0; swr=1; 
end
if (quad == 4)

    sw1=0;sw2=0;sw3=0; sw4=pwm; swv=0; swr=1; 
end

== matlab function Fbridge_sim/Subsystem1/Subsystem/Subsystem7/MATLAB Function ==
  data: ref input; quad output; err input
function quad = fcn(ref,err)
quad =1;

if (ref>=0) && (err>=0)
    quad =1;
end

if (ref>=0) && (err<0)
    quad =2;
end

if (ref<0) && (err>=0)
    quad =3;
end

if (ref<0) && (err<0)
    quad =4;
end

end
